simulink model "w3_warplab_buffers"  (Simulink 7.7)
settings: Solver=VariableStepDiscrete  SolverMode=SingleTasking  StartTime=0.0  StopTime=200000  RelTol=1e-3
InitFcn:
  | w3_warplab_buffers_init
StartFcn:
  | w3_warplab_buffers_init
values from neighbouring files (symbols this model uses):
  NumSamps_Rx_IQ = 2^15    (= 32768)    [w3_warplab_buffers_init.m]
  NumSamps_Rx_RSSI = 2^13    (= 8192)    [w3_warplab_buffers_init.m]
  NumSamps_Tx_IQ = 2^15    (= 32768)    [w3_warplab_buffers_init.m]
undefined symbols (not defined in the file or in its folder): gcbh, xlBlockLoadCallback, xlGetNormalizedPeriod
libraries: xbsIndex_r4 x1266, xbsEDKLib_r4 x1
(part 5 of 9)

== system w3_warplab_buffers/RSSI Clock Gen ==
  1LSB+0 : xbsIndex_r4/Slice  nbits=1  boolean_output=off  mode=Lower Bit Location + Width  bit1=0  base1=MSB of Input  bit0=0  base0=LSB of Input  dbl_ovrd=off  block_type=slice
  1LSB+1 : xbsIndex_r4/Slice  nbits=1  boolean_output=off  mode=Lower Bit Location + Width  bit1=0  base1=MSB of Input  bit0=1  base0=LSB of Input  dbl_ovrd=off  block_type=slice
  1LSB+2 : xbsIndex_r4/Slice  nbits=1  boolean_output=off  mode=Lower Bit Location + Width  bit1=0  base1=MSB of Input  bit0=2  base0=LSB of Input  dbl_ovrd=off  block_type=slice
  Mux : xbsIndex_r4/Mux  inputs=3  en=off  latency=0  precision=Full  arith_type=Unsigned  n_bits=16  bin_pt=14  quantization=Truncate  overflow=Wrap  dbl_ovrd=off  block_type=mux
  RSSI Clock Generator : xbsIndex_r4/Counter  cnt_type=Free Running  cnt_to=Inf  operation=Up  start_count=0  cnt_by_val=1  arith_type=Unsigned  n_bits=3  bin_pt=0  load_pin=off  rst=off  en=off  explicit_period=on  period=1  dbl_ovrd=off  use_behavioral_HDL=off  implementation=Fabric  use_rpm=off  block_type=counter
      settings: block_version=VER_STRING_GOES_HERE
  Clk : Outport
  wires:
  1LSB+2/1 -> Mux/4
  1LSB+1/1 -> Mux/3
  1LSB+0/1 -> Mux/2
  RSSI Clock Generator/1 -> 1LSB+0/1, 1LSB+1/1, 1LSB+2/1
  Mux/1 -> Clk/1
  [RSSI_CLK_SEL] -> Mux/1

== system w3_warplab_buffers/RX Start ==
  note: Block will condition the trigger input so that the RX state machine will only start when at least one buffer is enabled.
  Trigger In : Inport
  Logical5 : xbsIndex_r4/Logical  logical_function=OR  inputs=4  en=off  latency=0  precision=Full  arith_type=Unsigned  n_bits=16  bin_pt=0  align_bp=on  dbl_ovrd=off  block_type=logical
      settings: block_version=8.2
  Logical7 : xbsIndex_r4/Logical  logical_function=AND  inputs=2  en=off  latency=0  precision=Full  arith_type=Unsigned  n_bits=16  bin_pt=0  align_bp=on  dbl_ovrd=off  block_type=logical
      settings: block_version=8.2
  Posedge : Subsystem
  RX Start : Outport
  wires:
  [RFA_RX_BUF_EN] -> Logical5/1
  [RFB_RX_BUF_EN] -> Logical5/2
  [RFC_RX_BUF_EN] -> Logical5/3
  [RFD_RX_BUF_EN] -> Logical5/4
  Trigger In/1 -> Logical7/1
  Logical5/1 -> Logical7/2
  Logical7/1 -> Posedge/1(D)
  Posedge/1(Q) -> RX Start/1

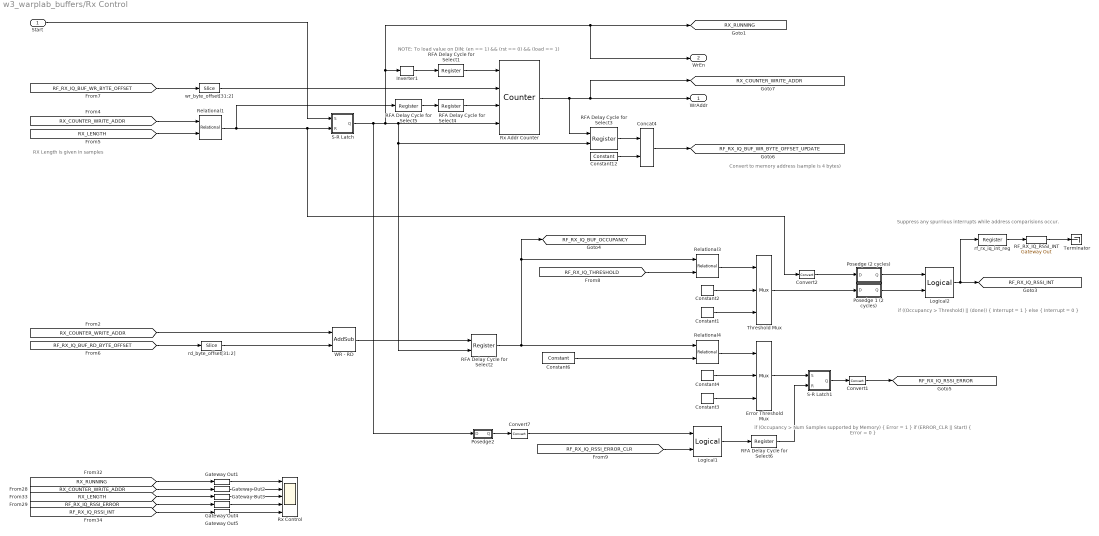
== system w3_warplab_buffers/Rx Control ==
  note: if ((Occupancy > Threshold) || (done)) {
      |     Interrupt = 1
      | } else {
      |     Interrupt = 0
      | }
  note: NOTE: To load value on DIN: (en == 1) && (rst == 0) && (load == 1)
  note: if (Occupancy > Num Samples supported by Memory) {
      |     Error = 1
      | }
      |
      | if (ERROR_CLR || Start) {
      |     Error = 0
      | }
  note: RX Length is given in samples
  note: Convert to memory address (sample is 4 bytes)
  note: Suppress any spurrious interrupts while
      | address comparisions occur.
  Start : Inport
  Concat4 : xbsIndex_r4/Concat  num_inputs=2  dbl_ovrd=off  block_type=concat
  Constant1 : xbsIndex_r4/Constant  const=1  gui_display_data_type=Fixed-point  arith_type=Unsigned  n_bits=1  bin_pt=0  preci_type=Single  exp_width=8  frac_width=24  explicit_period=off  period=1  equ=P=C  opselect=C  inp2=PCIN>>17  opr=+  inp1=P  carry=CIN  dbl_ovrd=off  block_type=constant
      settings: block_version=10.1.2
  Constant12 : xbsIndex_r4/Constant  const=0  gui_display_data_type=Fixed-point  arith_type=Unsigned  n_bits=2  bin_pt=0  preci_type=Single  exp_width=8  frac_width=24  explicit_period=off  period=1  equ=P=C  opselect=C  inp2=PCIN>>17  opr=+  inp1=P  carry=CIN  dbl_ovrd=off  block_type=constant
  Constant2 : xbsIndex_r4/Constant  const=0  gui_display_data_type=Fixed-point  arith_type=Unsigned  n_bits=1  bin_pt=0  preci_type=Single  exp_width=8  frac_width=24  explicit_period=off  period=1  equ=P=C  opselect=C  inp2=PCIN>>17  opr=+  inp1=P  carry=CIN  dbl_ovrd=off  block_type=constant
      settings: block_version=10.1.2
  Constant3 : xbsIndex_r4/Constant  const=1  gui_display_data_type=Fixed-point  arith_type=Unsigned  n_bits=1  bin_pt=0  preci_type=Single  exp_width=8  frac_width=24  explicit_period=off  period=1  equ=P=C  opselect=C  inp2=PCIN>>17  opr=+  inp1=P  carry=CIN  dbl_ovrd=off  block_type=constant
      settings: block_version=10.1.2
  Constant4 : xbsIndex_r4/Constant  const=0  gui_display_data_type=Fixed-point  arith_type=Unsigned  n_bits=1  bin_pt=0  preci_type=Single  exp_width=8  frac_width=24  explicit_period=off  period=1  equ=P=C  opselect=C  inp2=PCIN>>17  opr=+  inp1=P  carry=CIN  dbl_ovrd=off  block_type=constant
      settings: block_version=10.1.2
  Constant6 : xbsIndex_r4/Constant  const=NumSamps_Rx_IQ  gui_display_data_type=Fixed-point  arith_type=Unsigned  n_bits=30  bin_pt=0  preci_type=Single  exp_width=8  frac_width=24  explicit_period=off  period=1  equ=P=C  opselect=C  inp2=PCIN>>17  opr=+  inp1=P  carry=CIN  dbl_ovrd=off  block_type=constant
      settings: block_version=10.1.2
  Convert1 : xbsIndex_r4/Convert  gui_display_data_type=Fixed-point  arith_type=Unsigned  n_bits=1  bin_pt=0  float_type=Single  exp_bits=8  fraction_bits=24  quantization=Truncate  overflow=Wrap  en=off  latency=0  dbl_ovrd=off  pipeline=off  block_type=convert
      settings: block_version=10.1.2
  Convert2 : xbsIndex_r4/Convert  gui_display_data_type=Fixed-point  arith_type=Unsigned  n_bits=1  bin_pt=0  float_type=Single  exp_bits=8  fraction_bits=24  quantization=Truncate  overflow=Wrap  en=off  latency=0  dbl_ovrd=off  pipeline=off  block_type=convert
      settings: block_version=10.1.2
  Convert7 : xbsIndex_r4/Convert  gui_display_data_type=Fixed-point  arith_type=Unsigned  n_bits=1  bin_pt=0  float_type=Single  exp_bits=8  fraction_bits=24  quantization=Truncate  overflow=Wrap  en=off  latency=0  dbl_ovrd=off  pipeline=off  block_type=convert
  Error Threshold Mux : xbsIndex_r4/Mux  inputs=2  en=off  latency=0  precision=Full  arith_type=Unsigned  n_bits=16  bin_pt=14  quantization=Truncate  overflow=Wrap  dbl_ovrd=off  block_type=mux
  Gateway Out{1..5} (5 alike) : xbsIndex_r4/Gateway Out  inherit_from_input=off  hdl_port=off  timing_constraint=None  locs_specified=off  LOCs={}  UseAsDAC=off  DACChannel='1'  block_type=gatewayout
      settings: infoedit="Gateway out block.  Converts Xilinx fixed point inputs into ouputs of type Simulink integer, double, or fixed point.<P><P>Hardware notes:  In hardware these blocks become top level output ports or are discarded, depending on how they are configured."  block_version=10.1.2
  Inverter1 : xbsIndex_r4/Inverter  en=off  latency=0  dbl_ovrd=off  block_type=inv
      settings: block_version=8.2
  Logical1 : xbsIndex_r4/Logical  logical_function=OR  inputs=2  en=off  latency=0  precision=Full  arith_type=Unsigned  n_bits=16  bin_pt=0  align_bp=on  dbl_ovrd=off  block_type=logical
  Logical2 : xbsIndex_r4/Logical  logical_function=OR  inputs=2  en=off  latency=0  precision=Full  arith_type=Unsigned  n_bits=16  bin_pt=0  align_bp=on  dbl_ovrd=off  block_type=logical
  Posedge (2 cycles) : Subsystem
  Posedge 1 (2 cycles) : Subsystem
  Posedge2 : Subsystem
  RFA Delay Cycle for Select{1,4..6} (4 alike) : xbsIndex_r4/Register  init=0  rst=off  en=off  dbl_ovrd=off  block_type=register
  RFA Delay Cycle for Select2 : xbsIndex_r4/Register  init=0  rst=off  en=on  dbl_ovrd=off  block_type=register
  RFA Delay Cycle for Select3 : xbsIndex_r4/Register  init=0  rst=off  en=on  dbl_ovrd=off  block_type=register
  RF_RX_IQ_RSSI_INT : xbsIndex_r4/Gateway Out  inherit_from_input=off  hdl_port=on  timing_constraint=None  locs_specified=off  LOCs={}  UseAsDAC=off  DACChannel='1'  block_type=gatewayout
      settings: block_version=8.2
  Relational1 : xbsIndex_r4/Relational  mode=a>=b  en=off  latency=0  dbl_ovrd=off  block_type=relational
      settings: block_version=8.2
  Relational3 : xbsIndex_r4/Relational  mode=a>b  en=off  latency=0  dbl_ovrd=off  block_type=relational
      settings: block_version=8.2
  Relational4 : xbsIndex_r4/Relational  mode=a>b  en=off  latency=0  dbl_ovrd=off  block_type=relational
      settings: block_version=8.2
  Rx Addr Counter : xbsIndex_r4/Counter  cnt_type=Free Running  cnt_to=Inf  operation=Up  start_count=0  cnt_by_val=1  arith_type=Unsigned  n_bits=30  bin_pt=0  load_pin=on  rst=on  en=on  explicit_period=off  period=1  dbl_ovrd=off  use_behavioral_HDL=off  implementation=Fabric  use_rpm=off  block_type=counter
      settings: block_version=8.2
  Rx Control : Scope  NumInputPorts=5
      settings: TimeRange=70000  YMin=0~0~0~0~0  YMax=1~1~1~100~20000
  S-R Latch : Subsystem
  S-R Latch1 : Subsystem
  Terminator : Terminator
  Threshold Mux : xbsIndex_r4/Mux  inputs=2  en=off  latency=0  precision=Full  arith_type=Unsigned  n_bits=16  bin_pt=14  quantization=Truncate  overflow=Wrap  dbl_ovrd=off  block_type=mux
  WR - RD : xbsIndex_r4/AddSub  mode=Subtraction  use_carryin=off  use_carryout=off  en=off  latency=0  precision=User Defined  arith_type=Unsigned  n_bits=30  bin_pt=0  quantization=Truncate  overflow=Wrap  dbl_ovrd=off  use_behavioral_HDL=off  hw_selection=Fabric  pipelined=off  block_type=addsub
  rd_byte_offset[31:2] : xbsIndex_r4/Slice  nbits=30  boolean_output=off  mode=Lower Bit Location + Width  bit1=0  base1=MSB of Input  bit0=2  base0=LSB of Input  dbl_ovrd=off  block_type=slice
  rf_rx_iq_int_reg : xbsIndex_r4/Register  init=0  rst=off  en=off  dbl_ovrd=off  block_type=register
  wr_byte_offset[31:2] : xbsIndex_r4/Slice  nbits=30  boolean_output=off  mode=Lower Bit Location + Width  bit1=0  base1=MSB of Input  bit0=2  base0=LSB of Input  dbl_ovrd=off  block_type=slice
  WrAddr : Outport
  WrEn : Outport  Port=2
  tag scope: RF_RX_IQ_BUF_OCCUPANCY=global, RF_RX_IQ_BUF_WR_BYTE_OFFSET_UPDATE=global, RF_RX_IQ_RSSI_ERROR=global, RF_RX_IQ_RSSI_INT=global, RX_COUNTER_WRITE_ADDR=global, RX_RUNNING=global
  wires:
  S-R Latch/1(Q) -> Inverter1/1, WrEn/1, [RX_RUNNING], Rx Addr Counter/4, RFA Delay Cycle for Select3/2, RFA Delay Cycle for Select2/2, Posedge2/1(D)
  Gateway Out5/1 -> Rx Control/5
  Gateway Out4/1 -> Rx Control/4
  Gateway Out3/1 -> Rx Control/3
  Gateway Out2/1 -> Rx Control/2
  Gateway Out1/1 -> Rx Control/1
  [RF_RX_IQ_BUF_RD_BYTE_OFFSET] -> rd_byte_offset[31:2]/1
  Relational3/1 -> Threshold Mux/1
  Constant1/1 -> Threshold Mux/3
  Constant2/1 -> Threshold Mux/2
  [RF_RX_IQ_THRESHOLD] -> Relational3/2
  Relational4/1 -> Error Threshold Mux/1
  Constant3/1 -> Error Threshold Mux/3
  Constant4/1 -> Error Threshold Mux/2
  Error Threshold Mux/1 -> S-R Latch1/1(S)
  Constant6/1 -> Relational4/2
  [RX_LENGTH] -> Relational1/2
  Relational1/1 -> RFA Delay Cycle for Select5/1, S-R Latch/2(R), Convert2/1
  Rx Addr Counter/1 -> [RX_COUNTER_WRITE_ADDR], WrAddr/1, RFA Delay Cycle for Select3/1
  Constant12/1 -> Concat4/2
  Concat4/1 -> [RF_RX_IQ_BUF_WR_BYTE_OFFSET_UPDATE]
  S-R Latch1/1(Q) -> Convert1/1
  Convert1/1 -> [RF_RX_IQ_RSSI_ERROR]
  [RF_RX_IQ_BUF_WR_BYTE_OFFSET] -> wr_byte_offset[31:2]/1
  wr_byte_offset[31:2]/1 -> Rx Addr Counter/2
  Inverter1/1 -> RFA Delay Cycle for Select1/1
  RFA Delay Cycle for Select1/1 -> Rx Addr Counter/1
  RF_RX_IQ_RSSI_INT/1 -> Terminator/1
  Logical1/1 -> RFA Delay Cycle for Select6/1
  [RF_RX_IQ_RSSI_ERROR_CLR] -> Logical1/2
  RFA Delay Cycle for Select3/1 -> Concat4/1
  RFA Delay Cycle for Select4/1 -> Rx Addr Counter/3
  RFA Delay Cycle for Select5/1 -> RFA Delay Cycle for Select4/1
  Logical2/1 -> [RF_RX_IQ_RSSI_INT], rf_rx_iq_int_reg/1
  Threshold Mux/1 -> Posedge 1 (2 cycles)/1(D)
  Convert2/1 -> Posedge (2 cycles)/1(D)
  [RX_COUNTER_WRITE_ADDR] -> Relational1/1
  [RX_COUNTER_WRITE_ADDR] -> WR - RD/1
  rd_byte_offset[31:2]/1 -> WR - RD/2
  WR - RD/1 -> RFA Delay Cycle for Select2/1
  RFA Delay Cycle for Select2/1 -> Relational4/1, [RF_RX_IQ_BUF_OCCUPANCY], Relational3/1
  Start/1 -> S-R Latch/1(S)
  RFA Delay Cycle for Select6/1 -> S-R Latch1/2(R)
  [RX_RUNNING] -> Gateway Out1/1
  [RX_COUNTER_WRITE_ADDR] -> Gateway Out2/1
  [RX_LENGTH] -> Gateway Out3/1
  [RF_RX_IQ_RSSI_ERROR] -> Gateway Out4/1
  [RF_RX_IQ_RSSI_INT] -> Gateway Out5/1
  Posedge 1 (2 cycles)/1(Q) -> Logical2/2
  Posedge (2 cycles)/1(Q) -> Logical2/1
  rf_rx_iq_int_reg/1 -> RF_RX_IQ_RSSI_INT/1
  Posedge2/1(Q) -> Convert7/1
  Convert7/1 -> Logical1/1

== system w3_warplab_buffers/TX Start ==
  note: Block will condition the trigger input so that the TX state machine will only start when at least one buffer is enabled.
  Trigger In : Inport
  Logical5 : xbsIndex_r4/Logical  logical_function=OR  inputs=4  en=off  latency=0  precision=Full  arith_type=Unsigned  n_bits=16  bin_pt=0  align_bp=on  dbl_ovrd=off  block_type=logical
      settings: block_version=8.2
  Logical7 : xbsIndex_r4/Logical  logical_function=AND  inputs=2  en=off  latency=0  precision=Full  arith_type=Unsigned  n_bits=16  bin_pt=0  align_bp=on  dbl_ovrd=off  block_type=logical
      settings: block_version=8.2
  Posedge : Subsystem
  TX Start : Outport
  wires:
  [RFA_TX_BUF_EN] -> Logical5/1
  [RFB_TX_BUF_EN] -> Logical5/2
  [RFC_TX_BUF_EN] -> Logical5/3
  [RFD_TX_BUF_EN] -> Logical5/4
  Trigger In/1 -> Logical7/1
  Logical5/1 -> Logical7/2
  Logical7/1 -> Posedge/1(D)
  Posedge/1(Q) -> TX Start/1

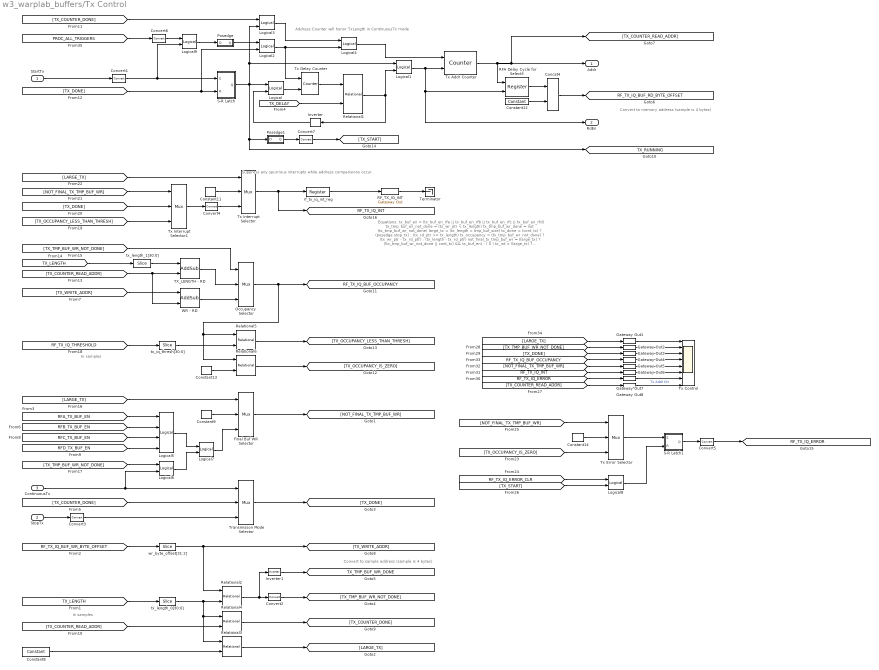
== system w3_warplab_buffers/Tx Control ==
  note: Address Counter will honor TxLength in ContinuousTx mode
  note: Convert to memory address (sample is 4 bytes)
  note: Convert to sample address (sample is 4 bytes)
  note: Equations:
      |   tx_buf_en               = (tx_buf_en_rfa || tx_buf_en_rfb || tx_buf_en_rfc || tx_buf_en_rfd)
      |
      |   tx_tmp_buf_wr_not_done  = (tx_wr_ptr < tx_length)
      |
      |   tx_tmp_buf_wr_done      = not (tx_tmp_buf_wr_not_done)
      |
      |   large_tx                = (tx_length > tmp_buf_size)
      |
      |   tx_done                 = (cont_tx) ? (posedge stop_tx) : (tx_rd_ptr >= tx_length)
      |
      |   tx_occupancy            = (tx_tmp_buf_wr_not_done) ? (tx_wr_ptr - tx_rd_ptr) : (tx_length - tx_rd_ptr)
      |
      |   not_final_tx_tmp_buf_wr = (large_tx) ? ((tx_tmp_buf_wr_not_done || cont_tx) && tx_buf_en) : ( 0 )
      |
      |   tx_int                  = (large_tx) ? ((not_final_tx_tmp_buf_wr) ? (tx_occupancy < tx_threshold) : tx_done) : ( 0 )
      |
      |   tx_err                  = (not_final_tx_tmp_buf_wr) ? (tx_occupancy == 0) : (0)
  note: In samples
  note: In samples
  note: Suppress any spurrious interrupts while
      | address comparisions occur.
  StartTx : Inport
  StopTx : Inport  Port=2
  ContinuousTx : Inport  Port=3
  Concat4 : xbsIndex_r4/Concat  num_inputs=2  dbl_ovrd=off  block_type=concat
  Constant11 : xbsIndex_r4/Constant  const=0  gui_display_data_type=Fixed-point  arith_type=Unsigned  n_bits=1  bin_pt=0  preci_type=Single  exp_width=8  frac_width=24  explicit_period=off  period=1  equ=P=C  opselect=C  inp2=PCIN>>17  opr=+  inp1=P  carry=CIN  dbl_ovrd=off  block_type=constant
      settings: block_version=10.1.2
  Constant12 : xbsIndex_r4/Constant  const=0  gui_display_data_type=Fixed-point  arith_type=Unsigned  n_bits=2  bin_pt=0  preci_type=Single  exp_width=8  frac_width=24  explicit_period=off  period=1  equ=P=C  opselect=C  inp2=PCIN>>17  opr=+  inp1=P  carry=CIN  dbl_ovrd=off  block_type=constant
  Constant13 : xbsIndex_r4/Constant  const=0  gui_display_data_type=Fixed-point  arith_type=Unsigned  n_bits=30  bin_pt=0  preci_type=Single  exp_width=8  frac_width=24  explicit_period=off  period=1  equ=P=C  opselect=C  inp2=PCIN>>17  opr=+  inp1=P  carry=CIN  dbl_ovrd=off  block_type=constant
      settings: block_version=10.1.2
  Constant14 : xbsIndex_r4/Constant  const=0  gui_display_data_type=Boolean  arith_type=Boolean  n_bits=1  bin_pt=0  preci_type=Single  exp_width=8  frac_width=24  explicit_period=off  period=1  equ=P=C  opselect=C  inp2=PCIN>>17  opr=+  inp1=P  carry=CIN  dbl_ovrd=off  block_type=constant
      settings: block_version=10.1.2
  Constant8 : xbsIndex_r4/Constant  const=NumSamps_Tx_IQ  gui_display_data_type=Fixed-point  arith_type=Unsigned  n_bits=30  bin_pt=0  preci_type=Single  exp_width=8  frac_width=24  explicit_period=off  period=1  equ=P=C  opselect=C  inp2=PCIN>>17  opr=+  inp1=P  carry=CIN  dbl_ovrd=off  block_type=constant
      settings: block_version=10.1.2
  Constant9 : xbsIndex_r4/Constant  const=0  gui_display_data_type=Fixed-point  arith_type=Unsigned  n_bits=1  bin_pt=0  preci_type=Single  exp_width=8  frac_width=24  explicit_period=off  period=1  equ=P=C  opselect=C  inp2=PCIN>>17  opr=+  inp1=P  carry=CIN  dbl_ovrd=off  block_type=constant
      settings: block_version=10.1.2
  Convert1 : xbsIndex_r4/Convert  gui_display_data_type=Fixed-point  arith_type=Boolean  n_bits=1  bin_pt=0  float_type=Single  exp_bits=8  fraction_bits=24  quantization=Truncate  overflow=Wrap  en=off  latency=0  dbl_ovrd=off  pipeline=off  block_type=convert
  Convert{2,4..5,7} (4 alike) : xbsIndex_r4/Convert  gui_display_data_type=Fixed-point  arith_type=Unsigned  n_bits=1  bin_pt=0  float_type=Single  exp_bits=8  fraction_bits=24  quantization=Truncate  overflow=Wrap  en=off  latency=0  dbl_ovrd=off  pipeline=off  block_type=convert
      Convert5 settings: block_version=10.1.2
  Convert3 : xbsIndex_r4/Convert  gui_display_data_type=Fixed-point  arith_type=Boolean  n_bits=1  bin_pt=0  float_type=Single  exp_bits=8  fraction_bits=24  quantization=Truncate  overflow=Wrap  en=off  latency=0  dbl_ovrd=off  pipeline=off  block_type=convert
  Convert6 : xbsIndex_r4/Convert  gui_display_data_type=Fixed-point  arith_type=Boolean  n_bits=1  bin_pt=0  float_type=Single  exp_bits=8  fraction_bits=24  quantization=Truncate  overflow=Wrap  en=off  latency=0  dbl_ovrd=off  pipeline=off  block_type=convert
  Final Buf WR  Selector : xbsIndex_r4/Mux  inputs=2  en=off  latency=0  precision=Full  arith_type=Unsigned  n_bits=16  bin_pt=14  quantization=Truncate  overflow=Wrap  dbl_ovrd=off  block_type=mux
      settings: block_version=9.1.01
  Gateway Out{1..8} (8 alike) : xbsIndex_r4/Gateway Out  inherit_from_input=off  hdl_port=off  timing_constraint=None  locs_specified=off  LOCs={}  UseAsDAC=off  DACChannel='1'  block_type=gatewayout
      settings: infoedit="Gateway out block.  Converts Xilinx fixed point inputs into ouputs of type Simulink integer, double, or fixed point.<P><P>Hardware notes:  In hardware these blocks become top level output ports or are discarded, depending on how they are configured."  block_version=10.1.2
  Inverter : xbsIndex_r4/Inverter  en=off  latency=0  dbl_ovrd=off  block_type=inv
      settings: block_version=8.2
  Inverter1 : xbsIndex_r4/Inverter  en=off  latency=0  dbl_ovrd=off  block_type=inv
      settings: block_version=8.2
  Logical{,1,3,7,9} (5 alike) : xbsIndex_r4/Logical  logical_function=AND  inputs=2  en=off  latency=0  precision=Full  arith_type=Unsigned  n_bits=16  bin_pt=0  align_bp=on  dbl_ovrd=off  block_type=logical
      settings: block_version=8.2
  Logical{2,4,6,8} (4 alike) : xbsIndex_r4/Logical  logical_function=OR  inputs=2  en=off  latency=0  precision=Full  arith_type=Unsigned  n_bits=16  bin_pt=0  align_bp=on  dbl_ovrd=off  block_type=logical
      Logical2 settings: block_version=8.2
      Logical6 settings: block_version=8.2
      Logical8 settings: block_version=8.2
  Logical5 : xbsIndex_r4/Logical  logical_function=OR  inputs=4  en=off  latency=0  precision=Full  arith_type=Unsigned  n_bits=16  bin_pt=0  align_bp=on  dbl_ovrd=off  block_type=logical
      settings: block_version=8.2
  Occupancy  Selector : xbsIndex_r4/Mux  inputs=2  en=off  latency=0  precision=Full  arith_type=Unsigned  n_bits=16  bin_pt=14  quantization=Truncate  overflow=Wrap  dbl_ovrd=off  block_type=mux
      settings: block_version=9.1.01
  Posedge : Subsystem
  Posedge1 : Subsystem
  RFA Delay Cycle for Select3 : xbsIndex_r4/Register  init=0  rst=off  en=on  dbl_ovrd=off  block_type=register
  RF_TX_IQ_INT : xbsIndex_r4/Gateway Out  inherit_from_input=off  hdl_port=on  timing_constraint=None  locs_specified=off  LOCs={}  UseAsDAC=off  DACChannel='1'  block_type=gatewayout
      settings: block_version=8.2
  Relational1 : xbsIndex_r4/Relational  mode=a>=b  en=off  latency=0  dbl_ovrd=off  block_type=relational
      settings: block_version=8.2
  Relational2 : xbsIndex_r4/Relational  mode=a<b  en=off  latency=0  dbl_ovrd=off  block_type=relational
      settings: block_version=8.2
  Relational3 : xbsIndex_r4/Relational  mode=a>b  en=off  latency=0  dbl_ovrd=off  block_type=relational
      settings: block_version=8.2
  Relational4 : xbsIndex_r4/Relational  mode=a<=b  en=off  latency=0  dbl_ovrd=off  block_type=relational
      settings: block_version=8.2
  Relational5 : xbsIndex_r4/Relational  mode=a<b  en=off  latency=0  dbl_ovrd=off  block_type=relational
      settings: block_version=8.2
  Relational6 : xbsIndex_r4/Relational  mode=a=b  en=off  latency=0  dbl_ovrd=off  block_type=relational
      settings: block_version=8.2
  S-R Latch : Subsystem
  S-R Latch1 : Subsystem
  TX_LENGTH - RD : xbsIndex_r4/AddSub  mode=Subtraction  use_carryin=off  use_carryout=off  en=off  latency=0  precision=User Defined  arith_type=Unsigned  n_bits=30  bin_pt=0  quantization=Truncate  overflow=Saturate  dbl_ovrd=off  use_behavioral_HDL=off  hw_selection=Fabric  pipelined=off  block_type=addsub
  Terminator : Terminator
  Transmisson Mode Selector : xbsIndex_r4/Mux  inputs=2  en=off  latency=0  precision=Full  arith_type=Unsigned  n_bits=16  bin_pt=14  quantization=Truncate  overflow=Wrap  dbl_ovrd=off  block_type=mux
      settings: block_version=9.1.01
  Tx Addr Counter : xbsIndex_r4/Counter  cnt_type=Free Running  cnt_to=Inf  operation=Up  start_count=0  cnt_by_val=1  arith_type=Unsigned  n_bits=30  bin_pt=0  load_pin=off  rst=on  en=on  explicit_period=off  period=1  dbl_ovrd=off  use_behavioral_HDL=off  implementation=Fabric  use_rpm=off  block_type=counter
      settings: block_version=8.2
  Tx Control : Scope  NumInputPorts=8
      settings: TimeRange=70000  YMin=0~0~0~0~0~0~0~0  YMax=2~1~1~1~1~100~1~20000  SaveName=ScopeData3
  Tx Delay Counter : xbsIndex_r4/Counter  cnt_type=Free Running  cnt_to=Inf  operation=Up  start_count=0  cnt_by_val=1  arith_type=Unsigned  n_bits=32  bin_pt=0  load_pin=off  rst=on  en=on  explicit_period=off  period=1  dbl_ovrd=off  use_behavioral_HDL=off  implementation=Fabric  use_rpm=off  block_type=counter
      settings: block_version=8.2
  Tx Error Selector : xbsIndex_r4/Mux  inputs=2  en=off  latency=0  precision=Full  arith_type=Unsigned  n_bits=16  bin_pt=14  quantization=Truncate  overflow=Wrap  dbl_ovrd=off  block_type=mux
      settings: block_version=9.1.01
  Tx Interrupt Selector : xbsIndex_r4/Mux  inputs=2  en=off  latency=0  precision=Full  arith_type=Unsigned  n_bits=16  bin_pt=14  quantization=Truncate  overflow=Wrap  dbl_ovrd=off  block_type=mux
      settings: block_version=9.1.01
  Tx Interrupt Selector1 : xbsIndex_r4/Mux  inputs=2  en=off  latency=0  precision=Full  arith_type=Unsigned  n_bits=16  bin_pt=14  quantization=Truncate  overflow=Wrap  dbl_ovrd=off  block_type=mux
      settings: block_version=9.1.01
  WR - RD : xbsIndex_r4/AddSub  mode=Subtraction  use_carryin=off  use_carryout=off  en=off  latency=0  precision=User Defined  arith_type=Unsigned  n_bits=30  bin_pt=0  quantization=Truncate  overflow=Saturate  dbl_ovrd=off  use_behavioral_HDL=off  hw_selection=Fabric  pipelined=off  block_type=addsub
  rf_tx_iq_int_reg : xbsIndex_r4/Register  init=0  rst=off  en=off  dbl_ovrd=off  block_type=register
  tx_iq_thresh[30:0] : xbsIndex_r4/Slice  nbits=30  boolean_output=off  mode=Lower Bit Location + Width  bit1=0  base1=MSB of Input  bit0=0  base0=LSB of Input  dbl_ovrd=off  block_type=slice
  tx_length_0[30:0] : xbsIndex_r4/Slice  nbits=30  boolean_output=off  mode=Lower Bit Location + Width  bit1=0  base1=MSB of Input  bit0=0  base0=LSB of Input  dbl_ovrd=off  block_type=slice
  tx_length_1[30:0] : xbsIndex_r4/Slice  nbits=30  boolean_output=off  mode=Lower Bit Location + Width  bit1=0  base1=MSB of Input  bit0=0  base0=LSB of Input  dbl_ovrd=off  block_type=slice
  wr_byte_offset[31:2] : xbsIndex_r4/Slice  nbits=30  boolean_output=off  mode=Lower Bit Location + Width  bit1=0  base1=MSB of Input  bit0=2  base0=LSB of Input  dbl_ovrd=off  block_type=slice
  Addr : Outport
  RdEn : Outport  Port=2
  tag scope: RF_TX_IQ_BUF_OCCUPANCY=global, RF_TX_IQ_BUF_RD_BYTE_OFFSET=global, RF_TX_IQ_ERROR=global, RF_TX_IQ_INT=global, TX_RUNNING=global, TX_TMP_BUF_WR_DONE=global
  wires:
  Tx Delay Counter/1 -> Relational1/1
  [TX_DELAY] -> Relational1/2
  StartTx/1 -> Convert1/1
  Logical/1 -> Tx Delay Counter/2
  S-R Latch/1(Q) -> Logical/1, Logical1/1, Logical3/2, [TX_RUNNING], Posedge1/1(D)
  Relational1/1 -> Inverter/1, Logical1/2
  Inverter/1 -> Logical/2
  Logical1/1 -> Tx Addr Counter/2, RdEn/1, RFA Delay Cycle for Select3/2
  Tx Addr Counter/1 -> Addr/1, RFA Delay Cycle for Select3/1, [TX_COUNTER_READ_ADDR]
  Logical2/1 -> Tx Delay Counter/1, Logical4/2
  Convert1/1 -> S-R Latch/1(S), Logical9/2
  Gateway Out5/1 -> Tx Control/5
  Gateway Out4/1 -> Tx Control/4
  Gateway Out3/1 -> Tx Control/3
  Gateway Out2/1 -> Tx Control/2
  Gateway Out1/1 -> Tx Control/1
  Gateway Out6/1 -> Tx Control/6
  Gateway Out7/1 -> Tx Control/7
  Gateway Out8/1 -> Tx Control/8  "Tx Addr Ctr"
  Logical3/1 -> Logical4/1
  Logical4/1 -> Tx Addr Counter/1
  Constant12/1 -> Concat4/2
  Concat4/1 -> [RF_TX_IQ_BUF_RD_BYTE_OFFSET]
  RFA Delay Cycle for Select3/1 -> Concat4/1
  [RF_TX_IQ_BUF_WR_BYTE_OFFSET] -> wr_byte_offset[31:2]/1
  wr_byte_offset[31:2]/1 -> Relational2/1, [TX_WRITE_ADDR]
  [TX_LENGTH] -> tx_length_0[30:0]/1
  Constant8/1 -> Relational3/2
  Relational3/1 -> [LARGE_TX]
  Relational2/1 -> Inverter1/1, Convert2/1
  Inverter1/1 -> [TX_TMP_BUF_WR_DONE]
  [TX_COUNTER_READ_ADDR] -> Relational4/2
  Relational4/1 -> [TX_COUNTER_DONE]
  [TX_COUNTER_DONE] -> Logical3/1
  ContinuousTx/1 -> Transmisson Mode Selector/1, Logical6/2
  StopTx/1 -> Convert3/1
  Convert3/1 -> Transmisson Mode Selector/3
  [TX_COUNTER_DONE] -> Transmisson Mode Selector/2
  Transmisson Mode Selector/1 -> [TX_DONE]
  [TX_DONE] -> S-R Latch/2(R), Logical2/2
  [TX_TMP_BUF_WR_NOT_DONE] -> Occupancy  Selector/1
  Occupancy  Selector/1 -> [RF_TX_IQ_BUF_OCCUPANCY], Relational5/1, Relational6/1
  [LARGE_TX] -> Final Buf WR  Selector/1
  [TX_LENGTH] -> tx_length_1[30:0]/1
  [TX_COUNTER_READ_ADDR] -> TX_LENGTH - RD/2, WR - RD/2
  [TX_WRITE_ADDR] -> WR - RD/1
  TX_LENGTH - RD/1 -> Occupancy  Selector/2
  WR - RD/1 -> Occupancy  Selector/3
  Constant9/1 -> Final Buf WR  Selector/2
  [TX_TMP_BUF_WR_NOT_DONE] -> Logical6/1
  [RFA_TX_BUF_EN] -> Logical5/1
  [RFB_TX_BUF_EN] -> Logical5/2
  [RFC_TX_BUF_EN] -> Logical5/3
  [RFD_TX_BUF_EN] -> Logical5/4
  Logical5/1 -> Logical7/1
  Logical6/1 -> Logical7/2
  Logical7/1 -> Final Buf WR  Selector/3
  Constant11/1 -> Tx Interrupt Selector/2
  Final Buf WR  Selector/1 -> [NOT_FINAL_TX_TMP_BUF_WR]
  Constant13/1 -> Relational6/2
  [RF_TX_IQ_THRESHOLD] -> tx_iq_thresh[30:0]/1
  Relational6/1 -> [TX_OCCUPANCY_IS_ZERO]
  Relational5/1 -> [TX_OCCUPANCY_LESS_THAN_THRESH]
  RF_TX_IQ_INT/1 -> Terminator/1
  [NOT_FINAL_TX_TMP_BUF_WR] -> Tx Interrupt Selector1/1
  [TX_DONE] -> Tx Interrupt Selector1/2
  [TX_OCCUPANCY_LESS_THAN_THRESH] -> Tx Interrupt Selector1/3
  [LARGE_TX] -> Tx Interrupt Selector/1
  Tx Interrupt Selector1/1 -> Convert4/1
  Tx Interrupt Selector/1 -> [RF_TX_IQ_INT], rf_tx_iq_int_reg/1
  Convert2/1 -> [TX_TMP_BUF_WR_NOT_DONE]
  Convert4/1 -> Tx Interrupt Selector/3
  [NOT_FINAL_TX_TMP_BUF_WR] -> Tx Error Selector/1
  [TX_OCCUPANCY_IS_ZERO] -> Tx Error Selector/3
  Constant14/1 -> Tx Error Selector/2
  S-R Latch1/1(Q) -> Convert5/1
  Convert5/1 -> [RF_TX_IQ_ERROR]
  Tx Error Selector/1 -> S-R Latch1/1(S)
  [RF_TX_IQ_ERROR_CLR] -> Logical8/1
  Logical8/1 -> S-R Latch1/2(R)
  [TX_START] -> Logical8/2
  [TX_COUNTER_READ_ADDR] -> Gateway Out8/1
  [LARGE_TX] -> Gateway Out1/1
  [TX_TMP_BUF_WR_NOT_DONE] -> Gateway Out2/1
  [TX_DONE] -> Gateway Out3/1
  [RF_TX_IQ_BUF_OCCUPANCY] -> Gateway Out4/1
  [NOT_FINAL_TX_TMP_BUF_WR] -> Gateway Out5/1
  [RF_TX_IQ_INT] -> Gateway Out6/1
  [RF_TX_IQ_ERROR] -> Gateway Out7/1
  tx_length_0[30:0]/1 -> Relational2/2, Relational3/1, Relational4/1
  tx_iq_thresh[30:0]/1 -> Relational5/2
  tx_length_1[30:0]/1 -> TX_LENGTH - RD/1
  rf_tx_iq_int_reg/1 -> RF_TX_IQ_INT/1
  Posedge/1(Q) -> Logical2/1
  Logical9/1 -> Posedge/1(D)
  [PROC_ALL_TRIGGERS] -> Convert6/1
  Posedge1/1(Q) -> Convert7/1
  Convert6/1 -> Logical9/1
  Convert7/1 -> [TX_START]

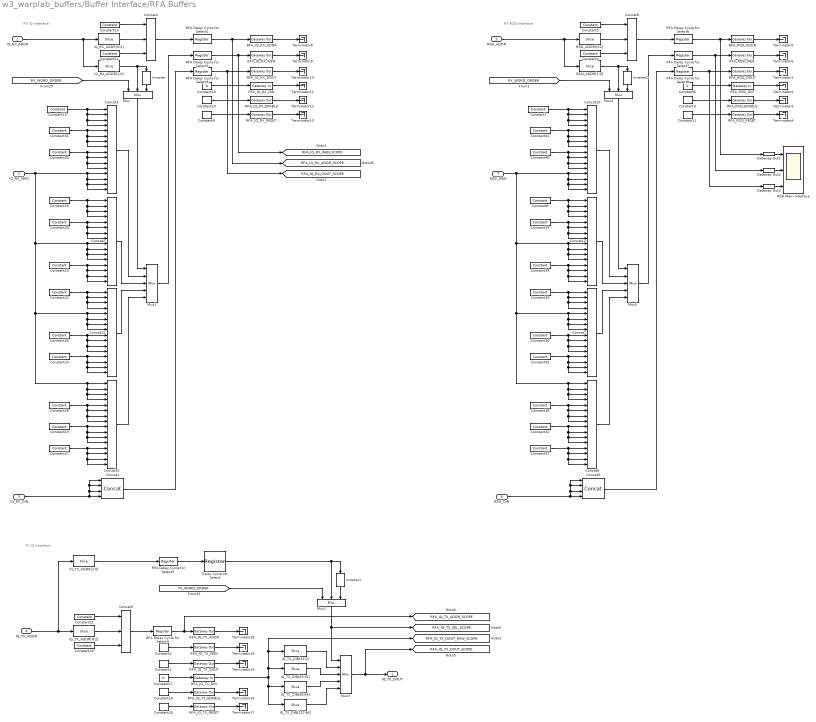
== system w3_warplab_buffers/Buffer Interface/RFA Buffers ==
  note: RX IQ Interface
  note: TX IQ Interface
  note: RX RSSI Interface
  IQ_RX_ADDR : Inport
  IQ_RX_WEN : Inport  Port=2
  IQ_RX_DIN : Inport  Port=3
  IQ_TX_ADDR : Inport  Port=4
  RSSI_ADDR : Inport  Port=5
  RSSI_DIN : Inport  Port=6
  RSSI_WEN : Inport  Port=7
  Concat1 : xbsIndex_r4/Concat  num_inputs=4  dbl_ovrd=off  block_type=concat
  Concat{2..3,6..7,10..13} (8 alike) : xbsIndex_r4/Concat  num_inputs=16  dbl_ovrd=off  block_type=concat
  Concat4 : xbsIndex_r4/Concat  num_inputs=3  dbl_ovrd=off  block_type=concat
  Concat5 : xbsIndex_r4/Concat  num_inputs=4  dbl_ovrd=off  block_type=concat
  Concat8 : xbsIndex_r4/Concat  num_inputs=3  dbl_ovrd=off  block_type=concat
  Concat9 : xbsIndex_r4/Concat  num_inputs=3  dbl_ovrd=off  block_type=concat
  Constant1 : xbsIndex_r4/Constant  const=0  gui_display_data_type=Fixed-point  arith_type=Unsigned  n_bits=128  bin_pt=0  preci_type=Single  exp_width=8  frac_width=24  explicit_period=off  period=1  equ=P=C  opselect=C  inp2=PCIN>>17  opr=+  inp1=P  carry=CIN  dbl_ovrd=off  block_type=constant
      settings: block_version=10.1.2
  Constant10 : xbsIndex_r4/Constant  const=1  gui_display_data_type=Boolean  arith_type=Boolean  n_bits=32  bin_pt=0  preci_type=Single  exp_width=8  frac_width=24  explicit_period=off  period=1  equ=P=C  opselect=C  inp2=PCIN>>17  opr=+  inp1=P  carry=CIN  dbl_ovrd=off  block_type=constant
      settings: block_version=10.1.2
  Constant11 : xbsIndex_r4/Constant  const=0  gui_display_data_type=Boolean  arith_type=Boolean  n_bits=32  bin_pt=0  preci_type=Single  exp_width=8  frac_width=24  explicit_period=off  period=1  equ=P=C  opselect=C  inp2=PCIN>>17  opr=+  inp1=P  carry=CIN  dbl_ovrd=off  block_type=constant
      settings: block_version=10.1.2
  Constant12 : xbsIndex_r4/Constant  const=0  gui_display_data_type=Fixed-point  arith_type=Unsigned  n_bits=4  bin_pt=0  preci_type=Single  exp_width=8  frac_width=24  explicit_period=off  period=1  equ=P=C  opselect=C  inp2=PCIN>>17  opr=+  inp1=P  carry=CIN  dbl_ovrd=off  block_type=constant
  Constant13 : xbsIndex_r4/Constant  const=0  gui_display_data_type=Fixed-point  arith_type=Unsigned  n_bits=30 - ceil(log2(NumSamps_Rx_IQ))  bin_pt=0  preci_type=Single  exp_width=8  frac_width=24  explicit_period=off  period=1  equ=P=C  opselect=C  inp2=PCIN>>17  opr=+  inp1=P  carry=CIN  dbl_ovrd=off  block_type=constant
  Constant14 : Constant  Value=0
  Constant{7..8,15..16,19,22..24,26..41} (24 alike) : xbsIndex_r4/Constant  const=0  gui_display_data_type=Boolean  arith_type=Boolean  n_bits=1  bin_pt=0  preci_type=Single  exp_width=8  frac_width=24  explicit_period=off  period=1  equ=P=C  opselect=C  inp2=PCIN>>17  opr=+  inp1=P  carry=CIN  dbl_ovrd=off  block_type=constant
  Constant17 : Constant  Value=0
  Constant18 : xbsIndex_r4/Constant  const=1  gui_display_data_type=Boolean  arith_type=Boolean  n_bits=32  bin_pt=0  preci_type=Single  exp_width=8  frac_width=24  explicit_period=off  period=1  equ=P=C  opselect=C  inp2=PCIN>>17  opr=+  inp1=P  carry=CIN  dbl_ovrd=off  block_type=constant
      settings: block_version=10.1.2
  Constant2 : xbsIndex_r4/Constant  const=0  gui_display_data_type=Fixed-point  arith_type=Unsigned  n_bits=16  bin_pt=0  preci_type=Single  exp_width=8  frac_width=24  explicit_period=off  period=1  equ=P=C  opselect=C  inp2=PCIN>>17  opr=+  inp1=P  carry=CIN  dbl_ovrd=off  block_type=constant
      settings: block_version=10.1.2
  Constant20 : xbsIndex_r4/Constant  const=0  gui_display_data_type=Fixed-point  arith_type=Unsigned  n_bits=4  bin_pt=0  preci_type=Single  exp_width=8  frac_width=24  explicit_period=off  period=1  equ=P=C  opselect=C  inp2=PCIN>>17  opr=+  inp1=P  carry=CIN  dbl_ovrd=off  block_type=constant
  Constant21 : xbsIndex_r4/Constant  const=0  gui_display_data_type=Fixed-point  arith_type=Unsigned  n_bits=30 - ceil(log2(NumSamps_Tx_IQ))  bin_pt=0  preci_type=Single  exp_width=8  frac_width=24  explicit_period=off  period=1  equ=P=C  opselect=C  inp2=PCIN>>17  opr=+  inp1=P  carry=CIN  dbl_ovrd=off  block_type=constant
  Constant25 : xbsIndex_r4/Constant  const=0  gui_display_data_type=Boolean  arith_type=Boolean  n_bits=32  bin_pt=0  preci_type=Single  exp_width=8  frac_width=24  explicit_period=off  period=1  equ=P=C  opselect=C  inp2=PCIN>>17  opr=+  inp1=P  carry=CIN  dbl_ovrd=off  block_type=constant
      settings: block_version=10.1.2
  Constant3 : xbsIndex_r4/Constant  const=1  gui_display_data_type=Boolean  arith_type=Boolean  n_bits=32  bin_pt=0  preci_type=Single  exp_width=8  frac_width=24  explicit_period=off  period=1  equ=P=C  opselect=C  inp2=PCIN>>17  opr=+  inp1=P  carry=CIN  dbl_ovrd=off  block_type=constant
      settings: block_version=10.1.2
  Constant4 : xbsIndex_r4/Constant  const=0  gui_display_data_type=Fixed-point  arith_type=Unsigned  n_bits=4  bin_pt=0  preci_type=Single  exp_width=8  frac_width=24  explicit_period=off  period=1  equ=P=C  opselect=C  inp2=PCIN>>17  opr=+  inp1=P  carry=CIN  dbl_ovrd=off  block_type=constant
  Constant5 : xbsIndex_r4/Constant  const=0  gui_display_data_type=Fixed-point  arith_type=Unsigned  n_bits=31 - ceil(log2(NumSamps_Rx_RSSI))  bin_pt=0  preci_type=Single  exp_width=8  frac_width=24  explicit_period=off  period=1  equ=P=C  opselect=C  inp2=PCIN>>17  opr=+  inp1=P  carry=CIN  dbl_ovrd=off  block_type=constant
  Constant6 : Constant  Value=0
  Constant9 : xbsIndex_r4/Constant  const=0  gui_display_data_type=Boolean  arith_type=Boolean  n_bits=32  bin_pt=0  preci_type=Single  exp_width=8  frac_width=24  explicit_period=off  period=1  equ=P=C  opselect=C  inp2=PCIN>>17  opr=+  inp1=P  carry=CIN  dbl_ovrd=off  block_type=constant
      settings: block_version=10.1.2
  Delay Cycle for Select : xbsIndex_r4/Register  init=0  rst=off  en=off  dbl_ovrd=off  block_type=register
  Gateway Out1 : xbsIndex_r4/Gateway Out  inherit_from_input=off  hdl_port=off  timing_constraint=None  locs_specified=off  LOCs={}  UseAsDAC=off  DACChannel='1'  block_type=gatewayout
      settings: infoedit="Gateway out block.  Converts Xilinx fixed point inputs into ouputs of type Simulink integer, double, or fixed point.<P><P>Hardware notes:  In hardware these blocks become top level output ports or are discarded, depending on how they are configured."  block_version=10.1.2
  Gateway Out2 : xbsIndex_r4/Gateway Out  inherit_from_input=off  hdl_port=off  timing_constraint=None  locs_specified=off  LOCs={}  UseAsDAC=off  DACChannel='1'  block_type=gatewayout
      settings: infoedit="Gateway out block.  Converts Xilinx fixed point inputs into ouputs of type Simulink integer, double, or fixed point.<P><P>Hardware notes:  In hardware these blocks become top level output ports or are discarded, depending on how they are configured."  block_version=10.1.2
  Gateway Out3 : xbsIndex_r4/Gateway Out  inherit_from_input=off  hdl_port=off  timing_constraint=None  locs_specified=off  LOCs={}  UseAsDAC=off  DACChannel='1'  block_type=gatewayout
      settings: infoedit="Gateway out block.  Converts Xilinx fixed point inputs into ouputs of type Simulink integer, double, or fixed point.<P><P>Hardware notes:  In hardware these blocks become top level output ports or are discarded, depending on how they are configured."  block_version=10.1.2
  IQ_RX_ADDR[1:0] : xbsIndex_r4/Slice  nbits=2  boolean_output=off  mode=Lower Bit Location + Width  bit1=0  base1=MSB of Input  bit0=0  base0=LSB of Input  dbl_ovrd=off  block_type=slice
  IQ_RX_ADDR[N:2] : xbsIndex_r4/Slice  nbits=ceil(log2(NumSamps_Rx_IQ)) - 2  boolean_output=off  mode=Lower Bit Location + Width  bit1=0  base1=MSB of Input  bit0=2  base0=LSB of Input  dbl_ovrd=off  block_type=slice
  IQ_TX_ADDR[1:0] : xbsIndex_r4/Slice  nbits=2  boolean_output=off  mode=Lower Bit Location + Width  bit1=0  base1=MSB of Input  bit0=0  base0=LSB of Input  dbl_ovrd=off  block_type=slice
  IQ_TX_ADDR[N:2] : xbsIndex_r4/Slice  nbits=ceil(log2(NumSamps_Tx_IQ)) - 2  boolean_output=off  mode=Lower Bit Location + Width  bit1=0  base1=MSB of Input  bit0=2  base0=LSB of Input  dbl_ovrd=off  block_type=slice
  IQ_TX_DIN[127:96] : xbsIndex_r4/Slice  nbits=32  boolean_output=off  mode=Lower Bit Location + Width  bit1=0  base1=MSB of Input  bit0=96  base0=LSB of Input  dbl_ovrd=off  block_type=slice
  IQ_TX_DIN[31:0] : xbsIndex_r4/Slice  nbits=32  boolean_output=off  mode=Lower Bit Location + Width  bit1=0  base1=MSB of Input  bit0=0  base0=LSB of Input  dbl_ovrd=off  block_type=slice
  IQ_TX_DIN[63:32] : xbsIndex_r4/Slice  nbits=32  boolean_output=off  mode=Lower Bit Location + Width  bit1=0  base1=MSB of Input  bit0=32  base0=LSB of Input  dbl_ovrd=off  block_type=slice
  IQ_TX_DIN[95:64] : xbsIndex_r4/Slice  nbits=32  boolean_output=off  mode=Lower Bit Location + Width  bit1=0  base1=MSB of Input  bit0=64  base0=LSB of Input  dbl_ovrd=off  block_type=slice
  Inverter : xbsIndex_r4/Inverter  en=off  latency=0  dbl_ovrd=off  block_type=inv
  Inverter1 : xbsIndex_r4/Inverter  en=off  latency=0  dbl_ovrd=off  block_type=inv
  Inverter2 : xbsIndex_r4/Inverter  en=off  latency=0  dbl_ovrd=off  block_type=inv
  Mux : xbsIndex_r4/Mux  inputs=2  en=off  latency=0  precision=Full  arith_type=Unsigned  n_bits=16  bin_pt=14  quantization=Truncate  overflow=Wrap  dbl_ovrd=off  block_type=mux
  Mux1 : xbsIndex_r4/Mux  inputs=4  en=off  latency=0  precision=Full  arith_type=Unsigned  n_bits=16  bin_pt=14  quantization=Truncate  overflow=Wrap  dbl_ovrd=off  block_type=mux
  Mux2 : xbsIndex_r4/Mux  inputs=2  en=off  latency=0  precision=Full  arith_type=Unsigned  n_bits=16  bin_pt=14  quantization=Truncate  overflow=Wrap  dbl_ovrd=off  block_type=mux
  Mux3 : xbsIndex_r4/Mux  inputs=4  en=off  latency=0  precision=Full  arith_type=Unsigned  n_bits=16  bin_pt=14  quantization=Truncate  overflow=Wrap  dbl_ovrd=off  block_type=mux
  Mux4 : xbsIndex_r4/Mux  inputs=2  en=off  latency=0  precision=Full  arith_type=Unsigned  n_bits=16  bin_pt=14  quantization=Truncate  overflow=Wrap  dbl_ovrd=off  block_type=mux
  Mux5 : xbsIndex_r4/Mux  inputs=4  en=off  latency=0  precision=Full  arith_type=Unsigned  n_bits=16  bin_pt=14  quantization=Truncate  overflow=Wrap  dbl_ovrd=off  block_type=mux
  RFA Delay Cycle for Select{1..8} (8 alike) : xbsIndex_r4/Register  init=0  rst=off  en=off  dbl_ovrd=off  block_type=register
  RFA_IQ_RX_ADDR : xbsIndex_r4/Gateway Out  inherit_from_input=off  hdl_port=on  timing_constraint=None  locs_specified=off  LOCs={}  UseAsDAC=off  DACChannel='1'  block_type=gatewayout
  RFA_IQ_RX_DIN : xbsIndex_r4/Gateway In  gui_display_data_type=Fixed-point  arith_type=Unsigned  n_bits=128  bin_pt=0  preci_type=Single  exp_width=8  frac_width=24  quantization="Round  (unbiased: +/- Inf)"  overflow=Saturate  period=1  dbl_ovrd=off  timing_constraint=None  locs_specified=off  LOCs={}  UseAsADC=off  ADCChannel='1'  inherit_from_input=off  hdl_port=on  block_type=gatewayin
  RFA_IQ_RX_DOUT : xbsIndex_r4/Gateway Out  inherit_from_input=off  hdl_port=on  timing_constraint=None  locs_specified=off  LOCs={}  UseAsDAC=off  DACChannel='1'  block_type=gatewayout
  RFA_IQ_RX_ENABLE : xbsIndex_r4/Gateway Out  inherit_from_input=off  hdl_port=on  timing_constraint=None  locs_specified=off  LOCs={}  UseAsDAC=off  DACChannel='1'  block_type=gatewayout
  RFA_IQ_RX_RESET : xbsIndex_r4/Gateway Out  inherit_from_input=off  hdl_port=on  timing_constraint=None  locs_specified=off  LOCs={}  UseAsDAC=off  DACChannel='1'  block_type=gatewayout
  RFA_IQ_RX_WEN : xbsIndex_r4/Gateway Out  inherit_from_input=off  hdl_port=on  timing_constraint=None  locs_specified=off  LOCs={}  UseAsDAC=off  DACChannel='1'  block_type=gatewayout
  RFA_IQ_TX_ADDR : xbsIndex_r4/Gateway Out  inherit_from_input=off  hdl_port=on  timing_constraint=None  locs_specified=off  LOCs={}  UseAsDAC=off  DACChannel='1'  block_type=gatewayout
  RFA_IQ_TX_DIN : xbsIndex_r4/Gateway In  gui_display_data_type=Fixed-point  arith_type=Unsigned  n_bits=128  bin_pt=0  preci_type=Single  exp_width=8  frac_width=24  quantization="Round  (unbiased: +/- Inf)"  overflow=Saturate  period=1  dbl_ovrd=off  timing_constraint=None  locs_specified=off  LOCs={}  UseAsADC=off  ADCChannel='1'  inherit_from_input=off  hdl_port=on  block_type=gatewayin
  RFA_IQ_TX_DOUT : xbsIndex_r4/Gateway Out  inherit_from_input=off  hdl_port=on  timing_constraint=None  locs_specified=off  LOCs={}  UseAsDAC=off  DACChannel='1'  block_type=gatewayout
  RFA_IQ_TX_ENABLE : xbsIndex_r4/Gateway Out  inherit_from_input=off  hdl_port=on  timing_constraint=None  locs_specified=off  LOCs={}  UseAsDAC=off  DACChannel='1'  block_type=gatewayout
  RFA_IQ_TX_RESET : xbsIndex_r4/Gateway Out  inherit_from_input=off  hdl_port=on  timing_constraint=None  locs_specified=off  LOCs={}  UseAsDAC=off  DACChannel='1'  block_type=gatewayout
  RFA_IQ_TX_WEN : xbsIndex_r4/Gateway Out  inherit_from_input=off  hdl_port=on  timing_constraint=None  locs_specified=off  LOCs={}  UseAsDAC=off  DACChannel='1'  block_type=gatewayout
  RFA_RSSI_ADDR : xbsIndex_r4/Gateway Out  inherit_from_input=off  hdl_port=on  timing_constraint=None  locs_specified=off  LOCs={}  UseAsDAC=off  DACChannel='1'  block_type=gatewayout
  RFA_RSSI_DIN : xbsIndex_r4/Gateway In  gui_display_data_type=Fixed-point  arith_type=Unsigned  n_bits=128  bin_pt=0  preci_type=Single  exp_width=8  frac_width=24  quantization="Round  (unbiased: +/- Inf)"  overflow=Saturate  period=1  dbl_ovrd=off  timing_constraint=None  locs_specified=off  LOCs={}  UseAsADC=off  ADCChannel='1'  inherit_from_input=off  hdl_port=on  block_type=gatewayin
  RFA_RSSI_DOUT : xbsIndex_r4/Gateway Out  inherit_from_input=off  hdl_port=on  timing_constraint=None  locs_specified=off  LOCs={}  UseAsDAC=off  DACChannel='1'  block_type=gatewayout
  RFA_RSSI_ENABLE : xbsIndex_r4/Gateway Out  inherit_from_input=off  hdl_port=on  timing_constraint=None  locs_specified=off  LOCs={}  UseAsDAC=off  DACChannel='1'  block_type=gatewayout
  RFA_RSSI_RESET : xbsIndex_r4/Gateway Out  inherit_from_input=off  hdl_port=on  timing_constraint=None  locs_specified=off  LOCs={}  UseAsDAC=off  DACChannel='1'  block_type=gatewayout
  RFA_RSSI_WEN : xbsIndex_r4/Gateway Out  inherit_from_input=off  hdl_port=on  timing_constraint=None  locs_specified=off  LOCs={}  UseAsDAC=off  DACChannel='1'  block_type=gatewayout
  RSSI Mem Interface : Scope  NumInputPorts=3
      settings: TimeRange=70000  YMin=0~0~0  YMax=1~1~1  SaveName=ScopeData6
  RSSI_ADDR[1:0] : xbsIndex_r4/Slice  nbits=2  boolean_output=off  mode=Lower Bit Location + Width  bit1=0  base1=MSB of Input  bit0=0  base0=LSB of Input  dbl_ovrd=off  block_type=slice
  RSSI_ADDR[N:2] : xbsIndex_r4/Slice  nbits=ceil(log2(NumSamps_Rx_RSSI)) - 3  boolean_output=off  mode=Lower Bit Location + Width  bit1=0  base1=MSB of Input  bit0=2  base0=LSB of Input  dbl_ovrd=off  block_type=slice
  Terminator{1..6,8..14,16..19} (17 alike) : Terminator
  IQ_TX_DOUT : Outport
  tag scope: RFA_IQ_RX_ADDR_SCOPE=global, RFA_IQ_RX_DOUT_SCOPE=global, RFA_IQ_RX_WEN_SCOPE=global, RFA_IQ_TX_ADDR_SCOPE=global, RFA_IQ_TX_DOUT_RAW_SCOPE=global, RFA_IQ_TX_DOUT_SCOPE=global, RFA_IQ_TX_SEL_SCOPE=global
  wires:
  IQ_RX_ADDR/1 -> IQ_RX_ADDR[1:0]/1, IQ_RX_ADDR[N:2]/1
  IQ_RX_DIN/1 -> Concat1/4, Concat1/3, Concat1/2, Concat1/1
  RFA_IQ_RX_ADDR/1 -> Terminator8/1
  RFA_IQ_RX_WEN/1 -> Terminator9/1
  RFA_IQ_RX_DOUT/1 -> Terminator10/1
  RFA_IQ_RX_ENABLE/1 -> Terminator12/1
  RFA_IQ_RX_RESET/1 -> Terminator13/1
  RFA_IQ_RX_DIN/1 -> Terminator11/1
  Constant9/1 -> RFA_IQ_RX_RESET/1
  Constant10/1 -> RFA_IQ_RX_ENABLE/1
  Constant14/1 -> RFA_IQ_RX_DIN/1
  Constant13/1 -> Concat4/1
  IQ_RX_ADDR[N:2]/1 -> Concat4/2
  Constant12/1 -> Concat4/3
  Concat4/1 -> RFA Delay Cycle for Select1/1
  Mux1/1 -> RFA Delay Cycle for Select2/1
  IQ_TX_ADDR/1 -> IQ_TX_ADDR[1:0]/1, IQ_TX_ADDR[N:2]/1
  RFA_IQ_TX_ADDR/1 -> Terminator18/1
  RFA_IQ_TX_WEN/1 -> Terminator19/1
  RFA_IQ_TX_DOUT/1 -> Terminator14/1
  RFA_IQ_TX_ENABLE/1 -> Terminator16/1
  RFA_IQ_TX_RESET/1 -> Terminator17/1
  Constant25/1 -> RFA_IQ_TX_RESET/1
  Constant18/1 -> RFA_IQ_TX_ENABLE/1
  Constant21/1 -> Concat9/1
  IQ_TX_ADDR[N:2]/1 -> Concat9/2
  Constant20/1 -> Concat9/3
  Concat9/1 -> RFA Delay Cycle for Select4/1
  Constant2/1 -> RFA_IQ_TX_WEN/1
  Constant1/1 -> RFA_IQ_TX_DOUT/1
  IQ_TX_ADDR[1:0]/1 -> RFA Delay Cycle for Select5/1
  RFA_IQ_TX_DIN/1 -> IQ_TX_DIN[63:32]/1, IQ_TX_DIN[31:0]/1, [RFA_IQ_TX_DOUT_RAW_SCOPE], IQ_TX_DIN[127:96]/1, IQ_TX_DIN[95:64]/1
  IQ_TX_DIN[31:0]/1 -> Mux3/2
  IQ_TX_DIN[63:32]/1 -> Mux3/3
  RFA Delay Cycle for Select1/1 -> RFA_IQ_RX_ADDR/1, [RFA_IQ_RX_ADDR_SCOPE]
  RFA Delay Cycle for Select2/1 -> RFA_IQ_RX_WEN/1, [RFA_IQ_RX_WEN_SCOPE]
  Constant17/1 -> RFA_IQ_TX_DIN/1
  RFA Delay Cycle for Select3/1 -> RFA_IQ_RX_DOUT/1, [RFA_IQ_RX_DOUT_SCOPE]
  Concat1/1 -> RFA Delay Cycle for Select3/1
  RFA Delay Cycle for Select4/1 -> RFA_IQ_TX_ADDR/1, [RFA_IQ_TX_ADDR_SCOPE]
  RFA Delay Cycle for Select5/1 -> Delay Cycle for Select/1
  IQ_RX_ADDR[1:0]/1 -> Inverter/1, Mux/2
  Inverter/1 -> Mux/3
  Mux/1 -> Mux1/1
  Inverter1/1 -> Mux2/3
  Delay Cycle for Select/1 -> Inverter1/1, Mux2/2
  Mux2/1 -> Mux3/1, [RFA_IQ_TX_SEL_SCOPE]
  [RX_WORD_ORDER] -> Mux/1
  Mux3/1 -> IQ_TX_DOUT/1, [RFA_IQ_TX_DOUT_SCOPE]
  RSSI_ADDR/1 -> RSSI_ADDR[1:0]/1, RSSI_ADDR[N:2]/1
  RFA_RSSI_ADDR/1 -> Terminator5/1
  RFA_RSSI_WEN/1 -> Terminator6/1
  RFA_RSSI_DOUT/1 -> Terminator1/1
  RFA_RSSI_ENABLE/1 -> Terminator3/1
  RFA_RSSI_RESET/1 -> Terminator4/1
  RFA_RSSI_DIN/1 -> Terminator2/1
  Constant11/1 -> RFA_RSSI_RESET/1
  Constant3/1 -> RFA_RSSI_ENABLE/1
  Constant6/1 -> RFA_RSSI_DIN/1
  Constant5/1 -> Concat8/1
  RSSI_ADDR[N:2]/1 -> Concat8/2
  Constant4/1 -> Concat8/3
  Concat8/1 -> RFA Delay Cycle for Select6/1
  RFA Delay Cycle for Select6/1 -> RFA_RSSI_ADDR/1, Gateway Out1/1
  RFA Delay Cycle for Select7/1 -> RFA_RSSI_WEN/1, Gateway Out2/1
  RFA Delay Cycle for Select8/1 -> RFA_RSSI_DOUT/1, Gateway Out3/1
  RSSI_ADDR[1:0]/1 -> Inverter2/1, Mux4/2
  Inverter2/1 -> Mux4/3
  Gateway Out1/1 -> RSSI Mem Interface/1
  Gateway Out2/1 -> RSSI Mem Interface/2
  Gateway Out3/1 -> RSSI Mem Interface/3
  Constant15/1 -> Concat3/1, Concat3/2, Concat3/3, Concat3/4
  IQ_RX_WEN/1 -> Concat3/13, Concat3/14, Concat3/15, Concat3/16, Concat2/9, Concat2/10, Concat2/11, Concat2/12, Concat11/5, Concat11/6, Concat11/7, Concat11/8, Concat10/1, Concat10/2, Concat10/3, Concat10/4
  Constant16/1 -> Concat2/1, Concat2/2, Concat2/3, Concat2/4
  Constant23/1 -> Concat2/13, Concat2/14, Concat2/15, Concat2/16
  Constant22/1 -> Concat11/3, Concat11/4, Concat11/2, Concat11/1
  Constant24/1 -> Concat11/15, Concat11/16, Concat11/14, Concat11/13
  Constant26/1 -> Concat11/11, Concat11/12, Concat11/10, Concat11/9
  Constant27/1 -> Concat10/15, Concat10/16, Concat10/14, Concat10/13
  Constant19/1 -> Concat10/11, Concat10/12, Concat10/10, Concat10/9
  Constant28/1 -> Concat10/7, Concat10/8, Concat10/6, Concat10/5
  Constant29/1 -> Concat2/7, Concat2/8, Concat2/6, Concat2/5
  Constant30/1 -> Concat3/11, Concat3/12, Concat3/10, Concat3/9
  Constant31/1 -> Concat3/7, Concat3/8, Concat3/6, Concat3/5
  Concat3/1 -> Mux1/2
  Concat2/1 -> Mux1/3
  Concat11/1 -> Mux1/4
  Concat10/1 -> Mux1/5
  [RX_WORD_ORDER] -> Mux4/1
  [TX_WORD_ORDER] -> Mux2/1
  RSSI_DIN/1 -> Concat5/4, Concat5/3, Concat5/2, Concat5/1
  Mux5/1 -> RFA Delay Cycle for Select7/1
  Concat5/1 -> RFA Delay Cycle for Select8/1
  Mux4/1 -> Mux5/1
  Constant7/1 -> Concat13/1, Concat13/2, Concat13/3, Concat13/4
  RSSI_WEN/1 -> Concat13/13, Concat13/14, Concat13/15, Concat13/16, Concat12/9, Concat12/10, Concat12/11, Concat12/12, Concat7/5, Concat7/6, Concat7/7, Concat7/8, Concat6/1, Concat6/2, Concat6/3, Concat6/4
  Constant8/1 -> Concat12/1, Concat12/2, Concat12/3, Concat12/4
  Constant34/1 -> Concat12/13, Concat12/14, Concat12/15, Concat12/16
  Constant33/1 -> Concat7/3, Concat7/4, Concat7/2, Concat7/1
  Constant35/1 -> Concat7/15, Concat7/16, Concat7/14, Concat7/13
  Constant36/1 -> Concat7/11, Concat7/12, Concat7/10, Concat7/9
  Constant37/1 -> Concat6/15, Concat6/16, Concat6/14, Concat6/13
  Constant32/1 -> Concat6/11, Concat6/12, Concat6/10, Concat6/9
  Constant38/1 -> Concat6/7, Concat6/8, Concat6/6, Concat6/5
  Constant39/1 -> Concat12/7, Concat12/8, Concat12/6, Concat12/5
  Constant40/1 -> Concat13/11, Concat13/12, Concat13/10, Concat13/9
  Constant41/1 -> Concat13/7, Concat13/8, Concat13/6, Concat13/5
  Concat13/1 -> Mux5/2
  Concat12/1 -> Mux5/3
  Concat7/1 -> Mux5/4
  Concat6/1 -> Mux5/5
  IQ_TX_DIN[95:64]/1 -> Mux3/4
  IQ_TX_DIN[127:96]/1 -> Mux3/5
